simulink model "truck"  (R2018b)
settings: Solver=ode1  StartTime=0.0  StopTime=t_stop  FixedStep=t_sample  RelTol=1e-3
PreLoadFcn:
  | hybrid_truck_script
values from neighbouring files (symbols this model uses):
  air_density_sea_level = 1.225    [hybrid_truck_script.m]
  constant_velocity = 60    [hybrid_truck_script.m]
  distance = 0.20    (= 0.2)    [hybrid_truck_script.m]
  drag_coeff = 0.65    [hybrid_truck_script.m]
  elevation = route.data(:,3)    [hybrid_truck_script.m]
  engine_torque = lbftToNm.*engine.data(:,1)    [hybrid_truck_script.m]
  frontal_area = 5.14    [hybrid_truck_script.m]
  fuel_map = (3.6e6/(engine_efficiency*fuel_LHV*fuel_density))*            (rps_axes'*torque_axes)    [hybrid_truck_script.m]
  g = 9.81    [hybrid_truck_script.m]
  gear_ratios = gearbox.data    [hybrid_truck_script.m]
  gearRatio_differential = 4.263    [hybrid_truck_script.m]
  gradients = (pi/400).*route.data(:,5)    [hybrid_truck_script.m]
  idling_speed_rad = idling_speed/rpsToRPM    (= 62.8318530718)    [hybrid_truck_script.m]
  idling_torque = interp1(engine_rpm(1:2),engine_torque(1:2),idling_speed,                   'linear','extrap')    [hybrid_truck_script.m]
  momentOfInertia_engine = 2.55    [hybrid_truck_script.m]
  momentOfInertia_wheel = 2.5    [hybrid_truck_script.m]
  mpsToKPH = 3.6    [hybrid_truck_script.m]
  radius_wheel = 0.46    [hybrid_truck_script.m]
  rolling_resistance = 0.008    [hybrid_truck_script.m]
  rps_axes = linspace(min(engine_rad),max(engine_rad),n)    [hybrid_truck_script.m]
  selection = number associated with the drive cycle (see    [drop_bars.m]    (also in hybrid_truck_script.m = listdlg('ListString', drive_cycle))
  shift_down_rpm = 850/rpsToRPM    (= 89.0117918517)    [hybrid_truck_script.m]
  shift_up_rpm = 1600/rpsToRPM    (= 167.551608191)    [hybrid_truck_script.m]
  t_sample = 0.1    [hybrid_truck_script.m]
  torque_axes = linspace(min(engine_torque),max(engine_torque),n)    [hybrid_truck_script.m]
  total_mass = mass_truck + mass_trailor    (= 39150)    [hybrid_truck_script.m]
libraries: autolibshared x1
settings Model: Creator=tumisang  LastModifiedBy=tumisang

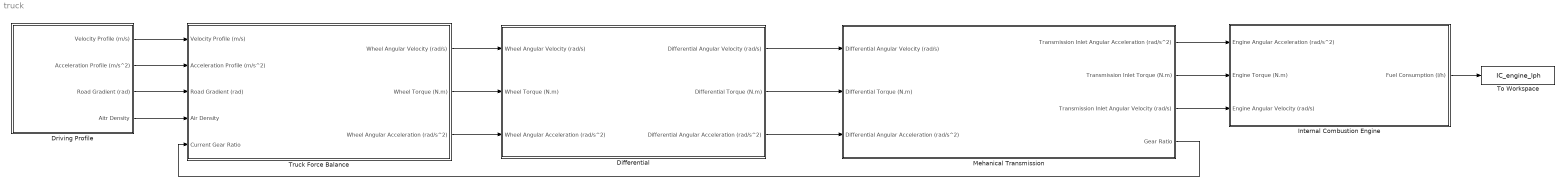
== system truck ==
  Differential : Subsystem
  Driving Profile : Subsystem
  Internal Combustion Engine : Subsystem
  Mehanical Transmission : Subsystem
  To Workspace : ToWorkspace  VariableName=IC_engine_lph  SaveFormat=Timeseries  SampleTime=-1
  Truck Force Balance : Subsystem
  wires:
  Truck Force Balance/1(Wheel Angular Velocity (rad/s)) -> Differential/1(Wheel Angular Velocity (rad/s))
  Truck Force Balance/3(Wheel Angular Acceleration (rad/s^2)) -> Differential/3(Wheel Angular Acceleration (rad/s^2))
  Differential/2(Differential Torque (N.m)) -> Mehanical Transmission/2(Differential Torque (N.m))
  Mehanical Transmission/3(Transmission Inlet Angular Velocity (rad/s)) -> Internal Combustion Engine/3(Engine Angular Velocity (rad/s))
  Differential/3(Differential Angular Acceleration (rad/s^2)) -> Mehanical Transmission/3(Differential Angular Acceleration (rad/s^2))
  Internal Combustion Engine/1(Fuel Consumption (l/h)) -> To Workspace/1
  Driving Profile/3(Road Gradient (rad)) -> Truck Force Balance/3(Road Gradient (rad))
  Truck Force Balance/2(Wheel Torque (N.m)) -> Differential/2(Wheel Torque (N.m))
  Mehanical Transmission/2(Transmission Inlet Torque (N.m)) -> Internal Combustion Engine/2(Engine Torque (N.m))
  Driving Profile/2(Acceleration Profile (m/s^2)) -> Truck Force Balance/2(Acceleration Profile (m/s^2))
  Mehanical Transmission/1(Transmission Inlet Angular Acceleration (rad/s^2)) -> Internal Combustion Engine/1(Engine Angular Acceleration (rad/s^2))
  Driving Profile/1(Velocity Profile (m/s)) -> Truck Force Balance/1(Velocity Profile (m/s))
  Mehanical Transmission/4(Gear Ratio) -> Truck Force Balance/5(Current Gear Ratio)
  Differential/1(Differential Angular Velocity (rad/s)) -> Mehanical Transmission/1(Differential Angular Velocity (rad/s))
  Driving Profile/4(Aitr Density) -> Truck Force Balance/4(Air Density)

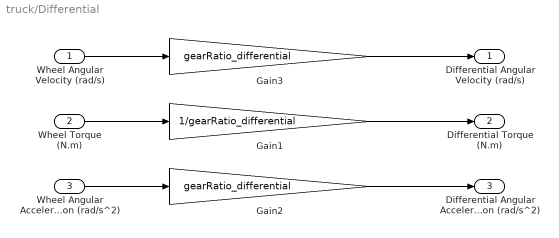
== system truck/Differential ==
  Wheel Angular Velocity (rad/s) : Inport
  Wheel Torque (N.m) : Inport  Port=2
  Wheel Angular Acceleration (rad/s^2) : Inport  Port=3
  Gain1 : Gain  Gain=1/gearRatio_differential
  Gain2 : Gain  Gain=gearRatio_differential
  Gain3 : Gain  Gain=gearRatio_differential
  Differential Angular Velocity (rad/s) : Outport
  Differential Torque (N.m) : Outport  Port=2
  Differential Angular Acceleration (rad/s^2) : Outport  Port=3
  wires:
  Gain2/1 -> Differential Angular Acceleration (rad/s^2)/1
  Gain3/1 -> Differential Angular Velocity (rad/s)/1
  Wheel Angular Acceleration (rad/s^2)/1 -> Gain2/1
  Wheel Torque (N.m)/1 -> Gain1/1
  Gain1/1 -> Differential Torque (N.m)/1
  Wheel Angular Velocity (rad/s)/1 -> Gain3/1

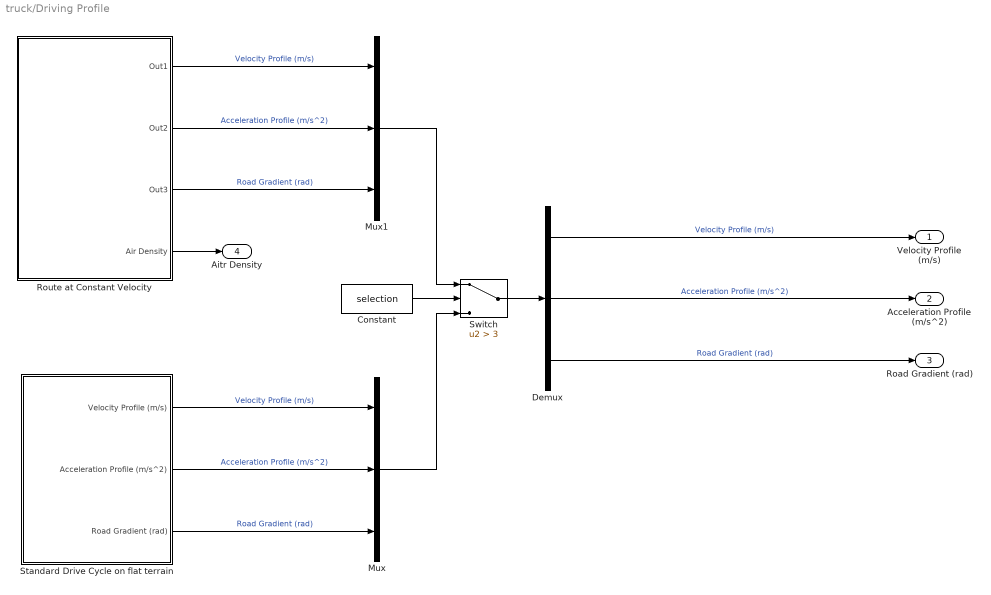
== system truck/Driving Profile ==
  Constant : Constant  Value=selection
  Demux : Demux  Outputs=3
  Mux : Mux  Inputs=3
  Mux1 : Mux  Inputs=3
  Route at Constant Velocity : Subsystem
  Standard Drive Cycle on flat terrain : Subsystem
  Switch : Switch  Criteria=u2 > Threshold  Threshold=3
  Velocity Profile (m/s) : Outport
  Acceleration Profile (m/s^2) : Outport  Port=2
  Road Gradient (rad) : Outport  Port=3
  Aitr Density : Outport  Port=4
  wires:
  Route at Constant Velocity/3(Out3) -> Mux1/3  "Road Gradient (rad)"
  Route at Constant Velocity/2(Out2) -> Mux1/2  "Acceleration Profile (m/s^2)"
  Demux/1 -> Velocity Profile (m/s)/1  "Velocity Profile (m/s)"
  Standard Drive Cycle on flat terrain/2(Acceleration Profile (m/s^2)) -> Mux/2  "Acceleration Profile (m/s^2)"
  Demux/2 -> Acceleration Profile (m/s^2)/1  "Acceleration Profile (m/s^2)"
  Standard Drive Cycle on flat terrain/3(Road Gradient (rad)) -> Mux/3  "Road Gradient (rad)"
  Demux/3 -> Road Gradient (rad)/1  "Road Gradient (rad)"
  Route at Constant Velocity/1(Out1) -> Mux1/1  "Velocity Profile (m/s)"
  Standard Drive Cycle on flat terrain/1(Velocity Profile (m/s)) -> Mux/1  "Velocity Profile (m/s)"
  Constant/1 -> Switch/2
  Switch/1 -> Demux/1
  Mux/1 -> Switch/3
  Mux1/1 -> Switch/1
  Route at Constant Velocity/4(Air Density) -> Aitr Density/1

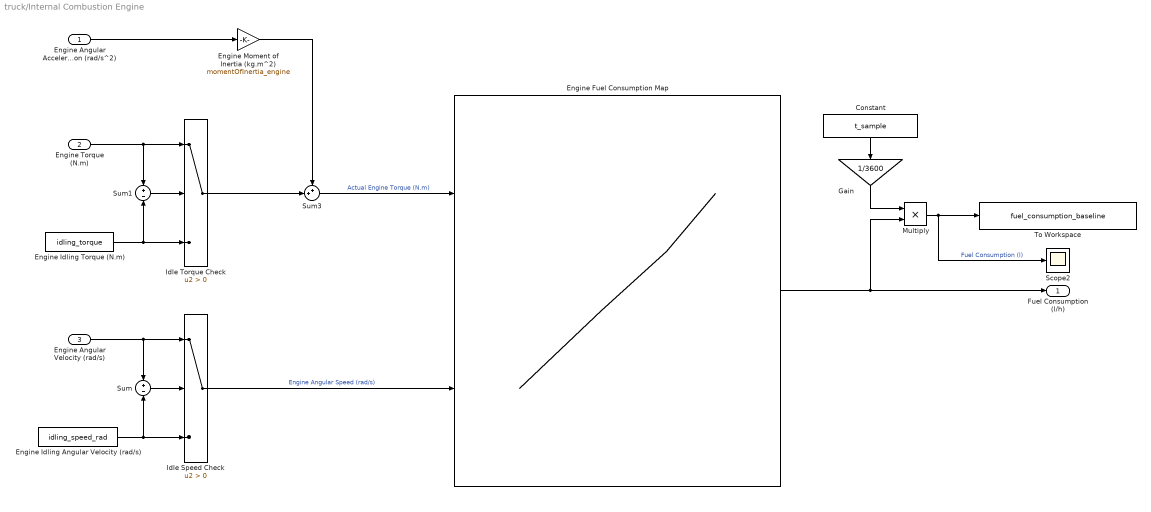
== system truck/Internal Combustion Engine ==
  Engine Angular Acceleration (rad/s^2) : Inport
  Engine Torque (N.m) : Inport  Port=2
  Engine Angular Velocity (rad/s) : Inport  Port=3
  Constant : Constant  Value=t_sample
  Engine Fuel Consumption Map : Lookup_n-D  BreakpointsForDimension1=torque_axes  BreakpointsForDimension2=rps_axes  Table=fuel_map  InternalRulePriority=Speed  RndMeth=Simplest  InputSameDT=on
  Engine Idling Angular Velocity (rad/s) : Constant  Value=idling_speed_rad
  Engine Idling Torque (N.m) : Constant  Value=idling_torque
  Engine Moment of Inertia (kg.m^2) : Gain  Gain=momentOfInertia_engine
  Gain : Gain  Gain=1/3600
  Idle Speed Check : Switch  Criteria=u2 > Threshold
  Idle Torque Check : Switch  Criteria=u2 > Threshold
  Multiply : Product
  Scope2 : Scope
  Sum : Sum  Inputs=+-
  Sum1 : Sum  Inputs=+-
  Sum3 : Sum  Inputs=++|
  To Workspace : ToWorkspace  VariableName=fuel_consumption_baseline  SaveFormat=Timeseries  SampleTime=-1
  Fuel Consumption (l/h) : Outport
  wires:
  Sum/1 -> Idle Speed Check/2
  Engine Idling Torque (N.m)/1 -> Idle Torque Check/3, Sum1/2
  Idle Speed Check/1 -> Engine Fuel Consumption Map/2  "Engine Angular Speed (rad/s)"
  Engine Idling Angular Velocity (rad/s)/1 -> Sum/2, Idle Speed Check/3
  Engine Torque (N.m)/1 -> Idle Torque Check/1, Sum1/1
  Sum1/1 -> Idle Torque Check/2
  Engine Angular Velocity (rad/s)/1 -> Sum/1, Idle Speed Check/1
  Sum3/1 -> Engine Fuel Consumption Map/1  "Actual Engine Torque (N.m)"
  Engine Angular Acceleration (rad/s^2)/1 -> Engine Moment of Inertia (kg.m^2)/1
  Engine Moment of Inertia (kg.m^2)/1 -> Sum3/1
  Engine Fuel Consumption Map/1 -> Fuel Consumption (l/h)/1, Multiply/2
  Idle Torque Check/1 -> Sum3/2
  Gain/1 -> Multiply/1
  Multiply/1 -> To Workspace/1, Scope2/1  "Fuel Consumption (l)"
  Constant/1 -> Gain/1

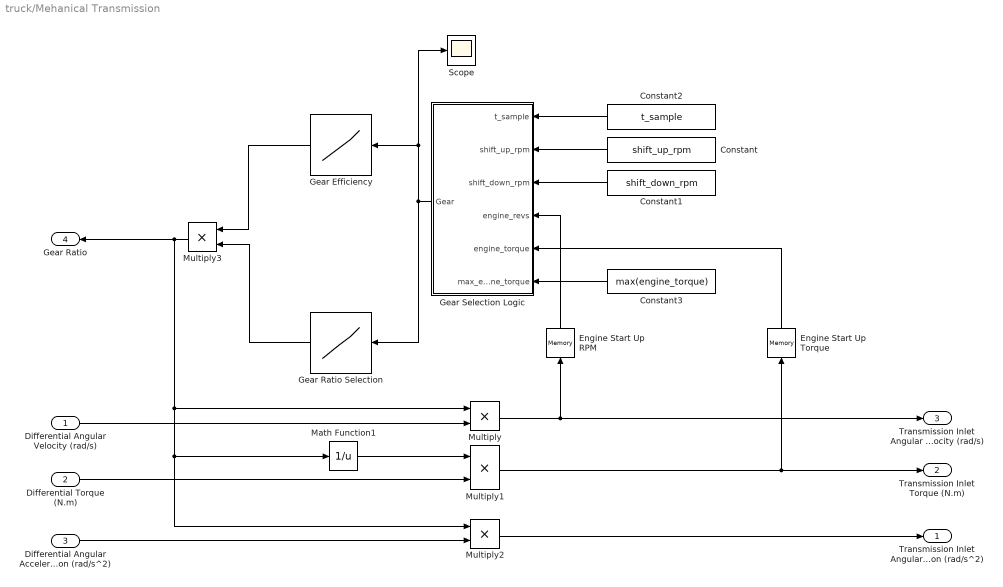
== system truck/Mehanical Transmission ==
  Differential Angular Velocity (rad/s) : Inport
  Differential Torque (N.m) : Inport  Port=2
  Differential Angular Acceleration (rad/s^2) : Inport  Port=3
  Constant : Constant  Value=shift_up_rpm
  Constant1 : Constant  Value=shift_down_rpm
  Constant2 : Constant  Value=t_sample
  Constant3 : Constant  Value=max(engine_torque)
  Engine Start Up RPM : Memory  InitialCondition=idling_speed_rad
  Engine Start Up Torque : Memory  InitialCondition=idling_torque
  Gear Efficiency : Lookup_n-D  NumberOfTableDimensions=1  BreakpointsForDimension1=gear_ratios(:,1)  BreakpointsForDimension2=[1:3]  Table=gear_ratios(:,3)  InternalRulePriority=Speed  RndMeth=Simplest  InputSameDT=on
  Gear Ratio Selection : Lookup_n-D  NumberOfTableDimensions=1  BreakpointsForDimension1=gear_ratios(:,1)  BreakpointsForDimension2=[1:3]  Table=gear_ratios(:,2)  InternalRulePriority=Speed  RndMeth=Simplest  InputSameDT=on
  Gear Selection Logic : Stateflow chart  TreatAsAtomicUnit=on
  Math Function1 : Math  Operator=reciprocal  SaturateOnIntegerOverflow=on
  Multiply{,1..3} (4 alike) : Product
  Scope : Scope
  Transmission Inlet Angular Acceleration (rad/s^2) : Outport
  Transmission Inlet Torque (N.m) : Outport  Port=2
  Transmission Inlet Angular Velocity (rad/s) : Outport  Port=3
  Gear Ratio : Outport  Port=4
  wires:
  Engine Start Up RPM/1 -> Gear Selection Logic/4(engine_revs)
  Gear Selection Logic/1(Gear) -> Gear Ratio Selection/1, Gear Efficiency/1, Scope/1
  Multiply1/1 -> Transmission Inlet Torque (N.m)/1, Engine Start Up Torque/1
  Gear Ratio Selection/1 -> Multiply3/2
  Multiply2/1 -> Transmission Inlet Angular Acceleration (rad/s^2)/1
  Math Function1/1 -> Multiply1/1
  Constant/1 -> Gear Selection Logic/2(shift_up_rpm)
  Constant1/1 -> Gear Selection Logic/3(shift_down_rpm)
  Differential Torque (N.m)/1 -> Multiply1/2
  Differential Angular Acceleration (rad/s^2)/1 -> Multiply2/2
  Differential Angular Velocity (rad/s)/1 -> Multiply/2
  Constant2/1 -> Gear Selection Logic/1(t_sample)
  Gear Efficiency/1 -> Multiply3/1
  Multiply3/1 -> Gear Ratio/1, Multiply/1, Multiply2/1, Math Function1/1
  Multiply/1 -> Engine Start Up RPM/1, Transmission Inlet Angular Velocity (rad/s)/1
  Constant3/1 -> Gear Selection Logic/6(max_engine_torque)
  Engine Start Up Torque/1 -> Gear Selection Logic/5(engine_torque)

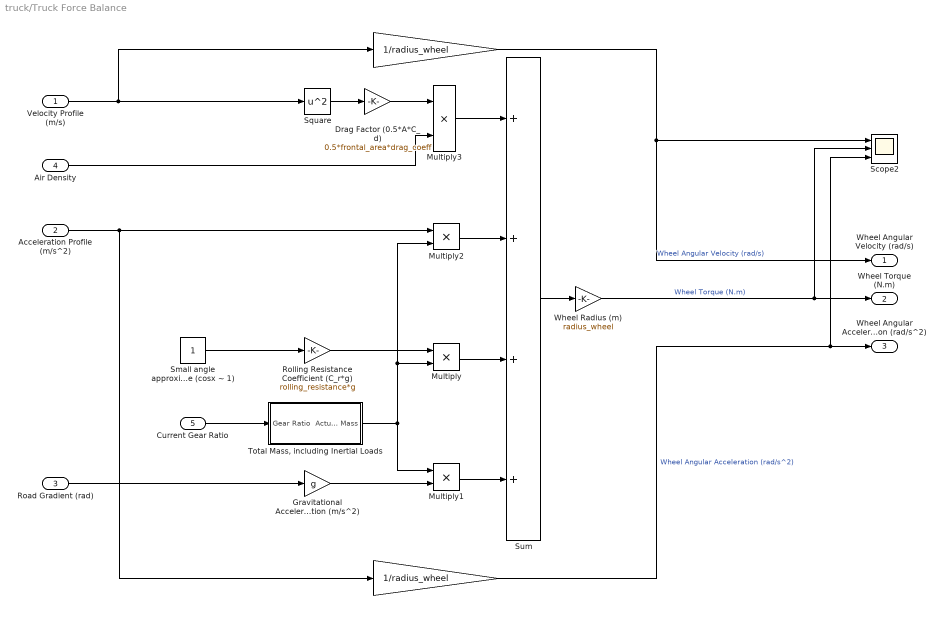
== system truck/Truck Force Balance ==
  Velocity Profile (m/s) : Inport
  Acceleration Profile (m/s^2) : Inport  Port=2
  Road Gradient (rad) : Inport  Port=3
  Air Density : Inport  Port=4
  Current Gear Ratio : Inport  Port=5
  " " : Gain  Gain=1/radius_wheel
  " " : Gain  Gain=1/radius_wheel
  Drag Factor (0.5*A*C_d) : Gain  Gain=0.5*frontal_area*drag_coeff
  Gravitational Acceleration (m/s^2) : Gain  Gain=g
  Multiply{,1..3} (4 alike) : Product
  Rolling Resistance Coefficient (C_r*g) : Gain  Gain=rolling_resistance*g
  Scope2 : Scope  NumInputPorts=3
  Small angle approximation for cosine (cosx ~ 1) : Constant
  Square : Math  Operator=square  SaturateOnIntegerOverflow=on
  Sum : Sum  Inputs=++++
  "Total Mass, including Inertial Loads" : Subsystem
  Wheel Radius (m) : Gain  Gain=radius_wheel
  Wheel Angular Velocity (rad/s) : Outport
  Wheel Torque (N.m) : Outport  Port=2
  Wheel Angular Acceleration (rad/s^2) : Outport  Port=3
  wires:
  Square/1 -> Drag Factor (0.5*A*C_d)/1
  Drag Factor (0.5*A*C_d)/1 -> Multiply3/1
  Road Gradient (rad)/1 -> Gravitational Acceleration (m/s^2)/1
  Gravitational Acceleration (m/s^2)/1 -> Multiply1/2
  Velocity Profile (m/s)/1 -> Square/1, " "/1
  Rolling Resistance Coefficient (C_r*g)/1 -> Multiply/1
  Sum/1 -> Wheel Radius (m)/1
  Wheel Radius (m)/1 -> Wheel Torque (N.m)/1, Scope2/2  "Wheel Torque (N.m)"
  " "/1 -> Scope2/3, Wheel Angular Acceleration (rad/s^2)/1  "Wheel Angular Acceleration (rad/s^2)"
  " "/1 -> Wheel Angular Velocity (rad/s)/1, Scope2/1  "Wheel Angular Velocity (rad/s)"
  Multiply2/1 -> Sum/2
  Small angle approximation for cosine (cosx ~ 1)/1 -> Rolling Resistance Coefficient (C_r*g)/1
  Acceleration Profile (m/s^2)/1 -> " "/1, Multiply2/1
  Current Gear Ratio/1 -> "Total Mass, including Inertial Loads"/1("Gear Ratio ")
  "Total Mass, including Inertial Loads"/1(Actual Mass) -> Multiply1/1, Multiply2/2, Multiply/2
  Multiply/1 -> Sum/3
  Multiply1/1 -> Sum/4
  Air Density/1 -> Multiply3/2
  Multiply3/1 -> Sum/1

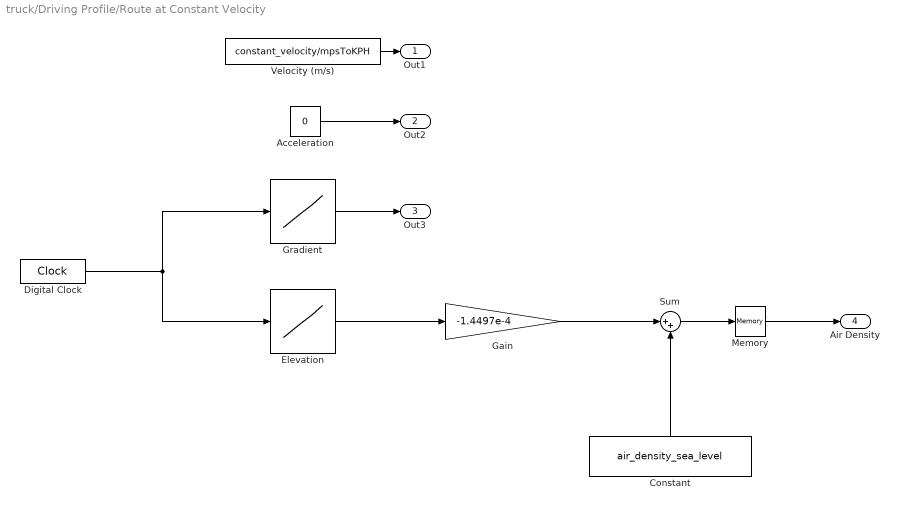
== system truck/Driving Profile/Route at Constant Velocity ==
  Acceleration : Constant  Value=0
  Constant : Constant  Value=air_density_sea_level
  Digital Clock : DigitalClock
  Elevation : Lookup_n-D  NumberOfTableDimensions=1  BreakpointsSpecification=Even spacing  BreakpointsForDimension1=distance(:,1)  Table=elevation  InternalRulePriority=Speed  RndMeth=Simplest  InputSameDT=on
  Gain : Gain  Gain=-1.4497e-4
  Gradient : Lookup_n-D  NumberOfTableDimensions=1  LookupTableObject=gradients  BreakpointsSpecification=Even spacing  BreakpointsForDimension1=linspace(0, max(distance), length(distance))  BreakpointsForDimension1FirstPoint=0  Table=gradients  InternalRulePriority=Speed  RndMeth=Simplest  InputSameDT=on
  Memory : Memory  InitialCondition=air_density_sea_level
  Sum : Sum  Inputs=|++
  Velocity (m/s) : Constant  Value=constant_velocity/mpsToKPH
  Out1 : Outport
  Out2 : Outport  Port=2
  Out3 : Outport  Port=3
  Air Density : Outport  Port=4
  wires:
  Acceleration/1 -> Out2/1
  Velocity (m/s)/1 -> Out1/1
  Gradient/1 -> Out3/1
  Elevation/1 -> Gain/1
  Gain/1 -> Sum/1
  Constant/1 -> Sum/2
  Sum/1 -> Memory/1
  Memory/1 -> Air Density/1
  Digital Clock/1 -> Gradient/1, Elevation/1

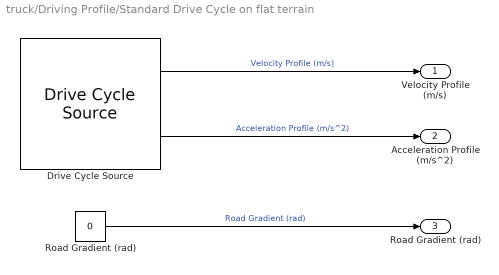
== system truck/Driving Profile/Standard Drive Cycle on flat terrain ==
  Drive Cycle Source : autolibshared/Drive Cycle Source  cycleVar=Heavy Heavy-Duty Diesel Truck (HHDDT) - Cruise Mode  fileVar=cycleFTP75.mat  tfinal="2083  seconds"  cycleRepeat=off  outAccPort=on  outGearPort=off  gearList=No gear data  t_wot1=5  xdot_woto=0  xdot_wot1=30  t_wot2=20  xdot_wot2=0  t_wotend=30  srcUnit=m/s  outUnit=m/s  srcAccUnit=m/s/s  outAccUnit=m/s^2  dt=t_sample  aMode=2
      settings: SourceProductName=Powertrain Blockset  SourceProductBaseCode=PW
  Road Gradient (rad) : Constant  Value=0
  Velocity Profile (m/s) : Outport
  Acceleration Profile (m/s^2) : Outport  Port=2
  Road Gradient (rad) : Outport  Port=3
  wires:
  Road Gradient (rad)/1 -> Road Gradient (rad)/1  "Road Gradient (rad)"
  Drive Cycle Source/1 -> Velocity Profile (m/s)/1  "Velocity Profile (m/s)"
  Drive Cycle Source/2 -> Acceleration Profile (m/s^2)/1  "Acceleration Profile (m/s^2)"

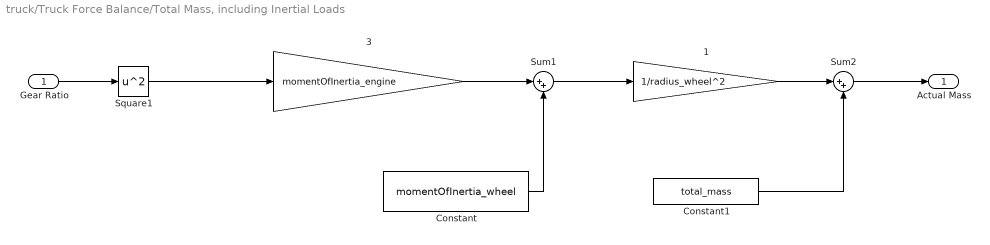
== system truck/Truck Force Balance/Total Mass, including Inertial Loads ==
  "Gear Ratio " : Inport
  " 1" : Gain  Gain=1/radius_wheel^2
  " 3" : Gain  Gain=momentOfInertia_engine
  Constant : Constant  Value=momentOfInertia_wheel
  Constant1 : Constant  Value=total_mass
  Square1 : Math  Operator=square  SaturateOnIntegerOverflow=on
  Sum1 : Sum  Inputs=|++
  Sum2 : Sum  Inputs=|++
  Actual Mass : Outport
  wires:
  Square1/1 -> " 3"/1
  Constant1/1 -> Sum2/2
  " 3"/1 -> Sum1/1
  Sum1/1 -> " 1"/1
  " 1"/1 -> Sum2/1
  "Gear Ratio "/1 -> Square1/1
  Constant/1 -> Sum1/2
  Sum2/1 -> Actual Mass/1

== stateflow chart truck/Mehanical Transmission/Gear Selection Logic ==
  settings: updateMethod=DISCRETE  sampleTime=t_sample
  state gear_state [parallel]
    settings: executionOrder=1
    state one
      entry:
      Gear = 1;
    state two
      entry:
      Gear = 2;
    state three
      entry:
      Gear = 3;
    state four
      entry:
      Gear = 4;
    state five
      entry:
      Gear = 5;
    state six
      entry:
      Gear = 6;
    state seven
      entry:
      Gear = 7;
    state eight
      entry:
      Gear = 8;
    state nine
      entry:
      Gear = 9;
    state ten
      entry:
      Gear = 10;
    state eleven
      entry:
      Gear = 11;
    state twelve
      entry:
      Gear = 12;
    state twelve1
      entry:
      Gear = 13;
    two -> three [order 1] : shift_up
    ten -> eleven [order 1] : shift_up
    one -> two : shift_up
    eleven -> twelve [order 1] : shift_up
    four -> five [order 1] : shift_up
    three -> four [order 1] : shift_up
    six -> seven [order 1] : shift_up
    (default) -> one
    nine -> ten [order 1] : shift_up
    five -> six [order 1] : shift_up
    seven -> eight [order 1] : shift_up
    twelve -> twelve1 [order 1] : shift_up
    eight -> nine [order 1] : shift_up
    two -> one [order 2] : shift_down
    three -> two [order 2] : shift_down
    four -> three [order 2] : shift_down
    five -> four [order 2] : shift_down
    six -> five [order 2] : shift_down
    seven -> six [order 2] : shift_down
    eight -> seven [order 2] : shift_down
    nine -> eight [order 2] : shift_down
    ten -> nine [order 2] : shift_down
    eleven -> ten [order 2] : shift_down
    twelve -> eleven [order 2] : shift_down
    twelve1 -> twelve : shift_down
  state selection_state [parallel]
    settings: executionOrder=2
    state steady_state
    state upshift
    state downshift
    (default) -> steady_state
    steady_state -> upshift [order 1] : after(t_sample*2,sec)
        | [engine_revs > shift_up_rpm && Gear < 13]
    steady_state -> downshift [order 2] : [(engine_revs < shift_down_rpm || engine_torque > max_engine_torque) && Gear > 1]
    downshift -> steady_state [order 1] : [engine_revs >= shift_down_rpm && engine_torque < max_engine_torque]
    downshift -> steady_state [order 2] : after(t_sample*2,sec)
        | [engine_revs < shift_down_rpm || engine_torque > max_engine_torque]
        | {gear_state.shift_down;}
    upshift -> steady_state [order 2] : after(t_sample*2,sec)
        | [engine_revs > shift_up_rpm]
        | {gear_state.shift_up;}
    upshift -> steady_state [order 1] : [engine_revs <= shift_up_rpm]
  data: t_sample input; Gear output double =1; gear_state local double; shift_up_rpm input double; shift_down_rpm input double; engine_revs input double; engine_torque input double; max_engine_torque input double
  data engine_revs settings: description=The engine angular velocity as determined by the previous gear ratio and the wheel velocity
  events: shift_up local FUNCTION_CALL_EVENT; shift_down local FUNCTION_CALL_EVENT
